simulink model "EBW_a1"  (Simulink 8.7)
settings: Solver=ode1  SolverMode=SingleTasking  StartTime=0.0  StopTime=500  FixedStep=0.001  RelTol=1e-3
(part 4 of 4)

== system EBW_a1/Veh_1_1/ComplexVehicleModel/Body and Tires/Body/Chassis Motion ==
  In1 : Inport
  Bus Creator : BusCreator  Inputs=54
  Demux : Demux  Outputs=54
  Out1 : Outport
  wires:
  Bus Creator/1 -> Out1/1
  Demux/54 -> Bus Creator/54  "ZO"
  Demux/53 -> Bus Creator/53  "ZCG_TM"
  Demux/52 -> Bus Creator/52  "ZCG_SM"
  Demux/51 -> Bus Creator/51  "YO"
  Demux/50 -> Bus Creator/50  "YCG_TM"
  Demux/49 -> Bus Creator/49  "YCG_SM"
  Demux/48 -> Bus Creator/48  "YAW"
  Demux/47 -> Bus Creator/47  "XO"
  Demux/46 -> Bus Creator/46  "XCG_TM"
  Demux/45 -> Bus Creator/45  "XCG_SM"
  Demux/44 -> Bus Creator/44  "VZ_SM"
  Demux/43 -> Bus Creator/43  "VZBF_SM"
  Demux/42 -> Bus Creator/42  "VZ"
  Demux/41 -> Bus Creator/41  "VY_SM"
  Demux/40 -> Bus Creator/40  "VYNF_SM"
  Demux/39 -> Bus Creator/39  "VYBF_SM"
  Demux/38 -> Bus Creator/38  "VY"
  Demux/37 -> Bus Creator/37  "VX_SM"
  Demux/36 -> Bus Creator/36  "VXNF_SM"
  Demux/35 -> Bus Creator/35  "VXBF_SM"
  Demux/34 -> Bus Creator/34  "VX"
  Demux/33 -> Bus Creator/33  "ROLL_E"
  Demux/32 -> Bus Creator/32  "ROLL"
  Demux/31 -> Bus Creator/31  "PITCH"
  Demux/30 -> Bus Creator/30  "KUG_STRR"
  Demux/29 -> Bus Creator/29  "KUG_GND"
  Demux/28 -> Bus Creator/28  "KSF_STRR"
  Demux/27 -> Bus Creator/27  "KSF_GND"
  Demux/26 -> Bus Creator/26  "BETAR"
  Demux/25 -> Bus Creator/25  "BETA"
  Demux/24 -> Bus Creator/24  "AZ_SM"
  Demux/23 -> Bus Creator/23  "AZBF_SM"
  Demux/22 -> Bus Creator/22  "AZ"
  Demux/21 -> Bus Creator/21  "AY_SM"
  Demux/20 -> Bus Creator/20  "AYNF_SM"
  Demux/19 -> Bus Creator/19  "AYG_SM"
  Demux/18 -> Bus Creator/18  "AYBF_SM"
  Demux/17 -> Bus Creator/17  "AY"
  Demux/16 -> Bus Creator/16  "AX_SM"
  Demux/15 -> Bus Creator/15  "AXNF_SM"
  Demux/14 -> Bus Creator/14  "AXBF_SM"
  Demux/13 -> Bus Creator/13  "AX"
  Demux/12 -> Bus Creator/12  "AV_Y"
  Demux/11 -> Bus Creator/11  "AV_R"
  Demux/10 -> Bus Creator/10  "AV_P"
  Demux/9 -> Bus Creator/9  "AVZ"
  Demux/8 -> Bus Creator/8  "AVY"
  Demux/7 -> Bus Creator/7  "AVX"
  Demux/6 -> Bus Creator/6  "AA_Y"
  Demux/5 -> Bus Creator/5  "AA_R"
  Demux/4 -> Bus Creator/4  "AA_P"
  Demux/3 -> Bus Creator/3  "AAZ"
  Demux/2 -> Bus Creator/2  "AAY"
  Demux/1 -> Bus Creator/1  "AAX"
  In1/1 -> Demux/1

== system EBW_a1/Veh_1_1/ComplexVehicleModel/Body and Tires/Body/Chassis States ==
  In1 : Inport
  Bus Creator : BusCreator  Inputs=24
  Demux : Demux  Outputs=24
  Out1 : Outport
  wires:
  In1/1 -> Demux/1
  Demux/1 -> Bus Creator/1  "q0"
  Demux/2 -> Bus Creator/2  "q1"
  Demux/3 -> Bus Creator/3  "q2"
  Demux/4 -> Bus Creator/4  "q3"
  Demux/5 -> Bus Creator/5  "q4"
  Demux/6 -> Bus Creator/6  "q5"
  Demux/7 -> Bus Creator/7  "q6"
  Demux/8 -> Bus Creator/8  "q7"
  Demux/9 -> Bus Creator/9  "u0"
  Demux/10 -> Bus Creator/10  "u1"
  Demux/11 -> Bus Creator/11  "u2"
  Demux/12 -> Bus Creator/12  "u3"
  Demux/13 -> Bus Creator/13  "u4"
  Demux/14 -> Bus Creator/14  "u5"
  Demux/15 -> Bus Creator/15  "u6"
  Demux/16 -> Bus Creator/16  "u7"
  Bus Creator/1 -> Out1/1  "Chassis States"
  Demux/17 -> Bus Creator/17  "up0"
  Demux/18 -> Bus Creator/18  "up1"
  Demux/19 -> Bus Creator/19  "up2"
  Demux/20 -> Bus Creator/20  "up3"
  Demux/21 -> Bus Creator/21  "up4"
  Demux/22 -> Bus Creator/22  "up5"
  Demux/23 -> Bus Creator/23  "up6"
  Demux/24 -> Bus Creator/24  "up7"

== system EBW_a1/Veh_1_1/ComplexVehicleModel/Body and Tires/Body/Wheel 1 ==
  In1 : Inport
  Bus Creator : BusCreator  Inputs=13
  Demux : Demux  Outputs=13
  Out1 : Outport
  wires:
  Bus Creator/1 -> Out1/1
  Demux/8 -> Bus Creator/8  "fy_whl"
  Demux/7 -> Bus Creator/7  "fx_whl"
  Demux/5 -> Bus Creator/5  "up0"
  Demux/4 -> Bus Creator/4  "u1"
  Demux/3 -> Bus Creator/3  "u0"
  Demux/2 -> Bus Creator/2  "q1"
  Demux/1 -> Bus Creator/1  "q0"
  In1/1 -> Demux/1
  Demux/6 -> Bus Creator/6  "up1"
  Demux/13 -> Bus Creator/13  "h_wc"
  Demux/12 -> Bus Creator/12  "mz_whl"
  Demux/11 -> Bus Creator/11  "my_whl"
  Demux/10 -> Bus Creator/10  "mx_whl"
  Demux/9 -> Bus Creator/9  "fz_whl"

== system EBW_a1/Veh_1_1/ComplexVehicleModel/Body and Tires/Body/Wheel 2 ==
  In1 : Inport
  Bus Creator : BusCreator  Inputs=13
  Demux : Demux  Outputs=13
  Out1 : Outport
  wires:
  Bus Creator/1 -> Out1/1
  Demux/8 -> Bus Creator/8  "fy_whl"
  Demux/7 -> Bus Creator/7  "fx_whl"
  Demux/5 -> Bus Creator/5  "up0"
  Demux/4 -> Bus Creator/4  "u1"
  Demux/3 -> Bus Creator/3  "u0"
  Demux/2 -> Bus Creator/2  "q1"
  Demux/1 -> Bus Creator/1  "q0"
  In1/1 -> Demux/1
  Demux/6 -> Bus Creator/6  "up1"
  Demux/13 -> Bus Creator/13  "h_wc"
  Demux/12 -> Bus Creator/12  "mz_whl"
  Demux/11 -> Bus Creator/11  "my_whl"
  Demux/10 -> Bus Creator/10  "mx_whl"
  Demux/9 -> Bus Creator/9  "fz_whl"

== system EBW_a1/Veh_1_1/ComplexVehicleModel/Body and Tires/Body/Wheel 3 ==
  In1 : Inport
  Bus Creator : BusCreator  Inputs=13
  Demux : Demux  Outputs=13
  Out1 : Outport
  wires:
  Bus Creator/1 -> Out1/1
  Demux/8 -> Bus Creator/8  "fy_whl"
  Demux/7 -> Bus Creator/7  "fx_whl"
  Demux/5 -> Bus Creator/5  "up0"
  Demux/4 -> Bus Creator/4  "u1"
  Demux/3 -> Bus Creator/3  "u0"
  Demux/2 -> Bus Creator/2  "q1"
  Demux/1 -> Bus Creator/1  "q0"
  In1/1 -> Demux/1
  Demux/6 -> Bus Creator/6  "up1"
  Demux/13 -> Bus Creator/13  "h_wc"
  Demux/12 -> Bus Creator/12  "mz_whl"
  Demux/11 -> Bus Creator/11  "my_whl"
  Demux/10 -> Bus Creator/10  "mx_whl"
  Demux/9 -> Bus Creator/9  "fz_whl"

== system EBW_a1/Veh_1_1/ComplexVehicleModel/Body and Tires/Body/Wheel 4 ==
  In1 : Inport
  Bus Creator : BusCreator  Inputs=13
  Demux : Demux  Outputs=13
  Out1 : Outport
  wires:
  Bus Creator/1 -> Out1/1
  Demux/8 -> Bus Creator/8  "fy_whl"
  Demux/7 -> Bus Creator/7  "fx_whl"
  Demux/5 -> Bus Creator/5  "up0"
  Demux/4 -> Bus Creator/4  "u1"
  Demux/3 -> Bus Creator/3  "u0"
  Demux/2 -> Bus Creator/2  "q1"
  Demux/1 -> Bus Creator/1  "q0"
  In1/1 -> Demux/1
  Demux/6 -> Bus Creator/6  "up1"
  Demux/13 -> Bus Creator/13  "h_wc"
  Demux/12 -> Bus Creator/12  "mz_whl"
  Demux/11 -> Bus Creator/11  "my_whl"
  Demux/10 -> Bus Creator/10  "mx_whl"
  Demux/9 -> Bus Creator/9  "fz_whl"

== system EBW_a1/Veh_1_1/ComplexVehicleModel/Body and Tires/Tires/Tires Force  2 ==
  In1 : Inport
  Bus Creator : BusCreator  Inputs=6
  Demux : Demux  Outputs=6
  Out1 : Outport
  wires:
  Bus Creator/1 -> Out1/1  "Tires_Forces"
  Demux/6 -> Bus Creator/6  "mz"
  Demux/5 -> Bus Creator/5  "my"
  Demux/4 -> Bus Creator/4  "mx"
  Demux/3 -> Bus Creator/3  "fz"
  In1/1 -> Demux/1
  Demux/2 -> Bus Creator/2  "fy"
  Demux/1 -> Bus Creator/1  "fx"

== system EBW_a1/Veh_1_1/ComplexVehicleModel/Body and Tires/Tires/Tires Force 1  ==
  In1 : Inport
  Bus Creator : BusCreator  Inputs=6
  Demux : Demux  Outputs=6
  Out1 : Outport
  wires:
  Demux/1 -> Bus Creator/1  "fx"
  Demux/2 -> Bus Creator/2  "fy"
  In1/1 -> Demux/1
  Demux/3 -> Bus Creator/3  "fz"
  Demux/4 -> Bus Creator/4  "mx"
  Demux/5 -> Bus Creator/5  "my"
  Demux/6 -> Bus Creator/6  "mz"
  Bus Creator/1 -> Out1/1  "Tires_Forces"

== system EBW_a1/Veh_1_1/ComplexVehicleModel/Body and Tires/Tires/Tires Force 3 ==
  In1 : Inport
  Bus Creator : BusCreator  Inputs=6
  Demux : Demux  Outputs=6
  Out1 : Outport
  wires:
  Demux/1 -> Bus Creator/1  "fx"
  Demux/2 -> Bus Creator/2  "fy"
  In1/1 -> Demux/1
  Demux/3 -> Bus Creator/3  "fz"
  Demux/4 -> Bus Creator/4  "mx"
  Demux/5 -> Bus Creator/5  "my"
  Demux/6 -> Bus Creator/6  "mz"
  Bus Creator/1 -> Out1/1  "Tires_Forces"

== system EBW_a1/Veh_1_1/ComplexVehicleModel/Body and Tires/Tires/Tires Force 4 ==
  In1 : Inport
  Bus Creator : BusCreator  Inputs=6
  Demux : Demux  Outputs=6
  Out1 : Outport
  wires:
  Bus Creator/1 -> Out1/1  "Tires_Forces"
  Demux/6 -> Bus Creator/6  "mz"
  Demux/5 -> Bus Creator/5  "my"
  Demux/4 -> Bus Creator/4  "mx"
  Demux/3 -> Bus Creator/3  "fz"
  In1/1 -> Demux/1
  Demux/2 -> Bus Creator/2  "fy"
  Demux/1 -> Bus Creator/1  "fx"

== system EBW_a1/Veh_1_1/ComplexVehicleModel/Body and Tires/Tires/Tires Force Ground ==
  In1 : Inport
  Bus Creator : BusCreator  Inputs=24
  Demux : Demux  Outputs=24
  Out1 : Outport
  wires:
  Demux/24 -> Bus Creator/24  "mz_gnd_r2"
  Demux/23 -> Bus Creator/23  "my_gnd_r2"
  Demux/22 -> Bus Creator/22  "mx_gnd_r2"
  Demux/21 -> Bus Creator/21  "fz_gnd_r2"
  Demux/20 -> Bus Creator/20  "fy_gnd_r2"
  Demux/19 -> Bus Creator/19  "fx_gnd_r2"
  Demux/18 -> Bus Creator/18  "mz_gnd_l2"
  Demux/17 -> Bus Creator/17  "my_gnd_l2"
  Demux/16 -> Bus Creator/16  "mx_gnd_l2"
  Demux/15 -> Bus Creator/15  "fz_gnd_l2"
  Demux/14 -> Bus Creator/14  "fy_gnd_l2"
  Demux/13 -> Bus Creator/13  "fx_gnd_l2"
  Demux/12 -> Bus Creator/12  "mz_gnd_r1"
  Demux/11 -> Bus Creator/11  "my_gnd_r1"
  Demux/10 -> Bus Creator/10  "mx_gnd_r1"
  Demux/9 -> Bus Creator/9  "fz_gnd_r1"
  Demux/8 -> Bus Creator/8  "fy_gnd_r1"
  Demux/7 -> Bus Creator/7  "fx_gnd_r1"
  Demux/1 -> Bus Creator/1  "fx_gnd_l1"
  Demux/2 -> Bus Creator/2  "fy_gnd_l1"
  In1/1 -> Demux/1
  Demux/3 -> Bus Creator/3  "fz_gnd_l1"
  Demux/4 -> Bus Creator/4  "mx_gnd_l1"
  Demux/5 -> Bus Creator/5  "my_gnd_l1"
  Demux/6 -> Bus Creator/6  "mz_gnd_l1"
  Bus Creator/1 -> Out1/1  "Tires_Forces"

== system EBW_a1/Veh_1_1/ComplexVehicleModel/Body and Tires/Tires/TiresStates ==
  In1 : Inport
  Bus Creator : BusCreator  Inputs=16
  Demux : Demux  Outputs=16
  Out1 : Outport
  wires:
  In1/1 -> Demux/1
  Demux/1 -> Bus Creator/1  "slip_lat_lf"
  Demux/2 -> Bus Creator/2  "slip_long_lf"
  Demux/3 -> Bus Creator/3  "slip_lat_rf"
  Demux/4 -> Bus Creator/4  "slip_long_rf"
  Demux/5 -> Bus Creator/5  "slip_lat_lr"
  Demux/6 -> Bus Creator/6  "slip_long_lr"
  Demux/7 -> Bus Creator/7  "slip_lat_rr"
  Demux/8 -> Bus Creator/8  "slip_long_rr"
  Demux/9 -> Bus Creator/9  "dslip_lat_lf"
  Demux/10 -> Bus Creator/10  "dslip_long_lf"
  Demux/11 -> Bus Creator/11  "dslip_lat_rf"
  Demux/12 -> Bus Creator/12  "dslip_long_rf"
  Demux/13 -> Bus Creator/13  "dslip_lat_lr"
  Demux/14 -> Bus Creator/14  "dslip_long_lr"
  Demux/15 -> Bus Creator/15  "dslip_lat_rr"
  Demux/16 -> Bus Creator/16  "dslip_long_rr"
  Bus Creator/1 -> Out1/1  "Tires_States"
